simulink model "KFPID"  (R2015a)
settings: Solver=ode4  StartTime=0.0  StopTime=10.0  FixedStep=0.01  RelTol=1e-3
libraries: simulink x4
settings Model: Creator=LAB425  LastModifiedBy=LAB425

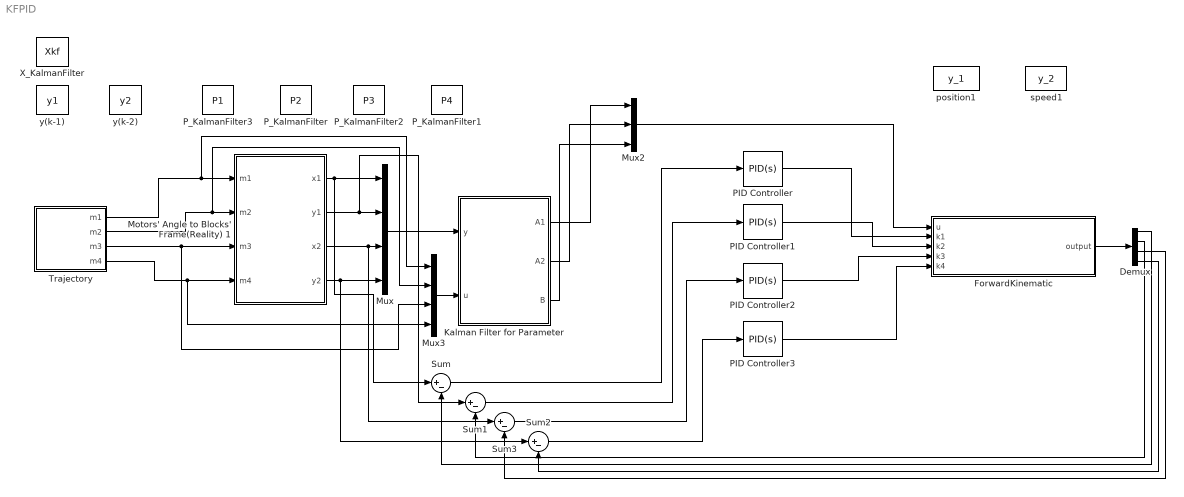
== system KFPID ==
  Demux : Demux
  ForwardKinematic : MATLAB Function  TreatAsAtomicUnit=on
  Kalman Filter for Parameter : MATLAB Function  TreatAsAtomicUnit=on
  Motors' Angle to Blocks' Frame(Reality) 1 : MATLAB Function  TreatAsAtomicUnit=on
  Mux : Mux
  Mux2 : Mux  Inputs=3
  Mux3 : Mux
  PID Controller{,1..3} (4 alike) : simulink/Continuous/PID Controller  Controller=PID  TimeDomain=Continuous-time  SampleTime=-1  IntegratorMethod=Forward Euler  FilterMethod=Forward Euler  Form=Parallel  UseFilter=on  ControllerParametersSource=internal  P=1  I=1  D=0  N=100  InitialConditionSource=internal  InitialConditionForIntegrator=0  InitialConditionForFilter=0  ExternalReset=none  LimitOutput=off  UpperSaturationLimit=inf  LowerSaturationLimit=-inf  LinearizeAsGain=on  AntiWindupMode=none  Kb=1  TrackingMode=off  Kt=1  PParamMin=[]  PParamMax=[]  IParamMin=[]  IParamMax=[]  DParamMin=[]  DParamMax=[]  NParamMin=[]  NParamMax=[]  KbParamMin=[]  KbParamMax=[]  KtParamMin=[]  KtParamMax=[]  POutMin=[]  POutMax=[]  IOutMin=[]  IOutMax=[]  DOutMin=[]  DOutMax=[]  NOutMin=[]  NOutMax=[]  KbOutMin=[]  KbOutMax=[]  KtOutMin=[]  KtOutMax=[]  IntegratorOutMin=[]  IntegratorOutMax=[]  FilterOutMin=[]  FilterOutMax=[]  SumOutMin=[]  SumOutMax=[]  SumI1OutMin=[]  SumI1OutMax=[]  SumI2OutMin=[]  SumI2OutMax=[]  SumI3OutMin=[]  SumI3OutMax=[]  SumDOutMin=[]  SumDOutMax=[]  SaturationOutMin=[]  SaturationOutMax=[]  IntegratorContinuousStateAttributes=''  IntegratorStateMustResolveToSignalObject=off  IntegratorRTWStateStorageClass=Auto  FilterContinuousStateAttributes=''  FilterStateMustResolveToSignalObject=off  FilterRTWStateStorageClass=Auto  DifferentiatorICPrevScaledInput=0  DifferentiatorOutMin=[]  DifferentiatorOutMax=[]
  P_KalmanFilter : DataStoreMemory  DataStoreName=P2  ReadBeforeWriteMsg=warning  WriteAfterWriteMsg=warning  WriteAfterReadMsg=warning  InitialValue=[0.001,0,0;0,0.002,0;0,0,0.001]  OutDataTypeStr=double
  P_KalmanFilter1 : DataStoreMemory  DataStoreName=P4  ReadBeforeWriteMsg=warning  WriteAfterWriteMsg=warning  WriteAfterReadMsg=warning  InitialValue=[0.001,0,0;0,0.002,0;0,0,0.001]  OutDataTypeStr=double
  P_KalmanFilter2 : DataStoreMemory  DataStoreName=P3  ReadBeforeWriteMsg=warning  WriteAfterWriteMsg=warning  WriteAfterReadMsg=warning  InitialValue=[0.001,0,0;0,0.002,0;0,0,0.001]  OutDataTypeStr=double
  P_KalmanFilter3 : DataStoreMemory  DataStoreName=P1  ReadBeforeWriteMsg=warning  WriteAfterWriteMsg=warning  WriteAfterReadMsg=warning  InitialValue=[0.001,0,0;0,0.002,0;0,0,0.001]  OutDataTypeStr=double
  Sum{,1..3} (4 alike) : Sum  Inputs=|+-
  Trajectory : Subsystem
  X_KalmanFilter : DataStoreMemory  DataStoreName=Xkf  ReadBeforeWriteMsg=warning  WriteAfterWriteMsg=warning  WriteAfterReadMsg=warning  InitialValue=[0,0,0,0;0,0,0,0;0,0,0,0]  OutDataTypeStr=double
  position1 : DataStoreMemory  DataStoreName=y_1  ReadBeforeWriteMsg=warning  WriteAfterWriteMsg=warning  WriteAfterReadMsg=warning  InitialValue=[0,0,0,0]  OutDataTypeStr=double
  speed1 : DataStoreMemory  DataStoreName=y_2  ReadBeforeWriteMsg=warning  WriteAfterWriteMsg=warning  WriteAfterReadMsg=warning  InitialValue=[0,0,0,0]  OutDataTypeStr=double
  y(k-1) : DataStoreMemory  DataStoreName=y1  ReadBeforeWriteMsg=warning  WriteAfterWriteMsg=warning  WriteAfterReadMsg=warning  InitialValue=[0,0,0,0]  OutDataTypeStr=double
  y(k-2) : DataStoreMemory  DataStoreName=y2  ReadBeforeWriteMsg=warning  WriteAfterWriteMsg=warning  WriteAfterReadMsg=warning  InitialValue=[0,0,0,0]  OutDataTypeStr=double
  wires:
  Motors' Angle to Blocks' Frame(Reality) 1/2(y1) -> Mux/2, Sum1/1
  Motors' Angle to Blocks' Frame(Reality) 1/3(x2) -> Sum3/1, Mux/3
  Motors' Angle to Blocks' Frame(Reality) 1/4(y2) -> Mux/4, Sum2/1
  Motors' Angle to Blocks' Frame(Reality) 1/1(x1) -> Mux/1, Sum/1
  Mux/1 -> Kalman Filter for Parameter/1(y)
  Mux3/1 -> Kalman Filter for Parameter/2(u)
  Trajectory/3(m3) -> Motors' Angle to Blocks' Frame(Reality) 1/3(m3), Mux3/3
  Trajectory/2(m2) -> Mux3/2, Motors' Angle to Blocks' Frame(Reality) 1/2(m2)
  Trajectory/4(m4) -> Motors' Angle to Blocks' Frame(Reality) 1/4(m4), Mux3/4
  Trajectory/1(m1) -> Mux3/1, Motors' Angle to Blocks' Frame(Reality) 1/1(m1)
  PID Controller/1 -> ForwardKinematic/2(k1)
  PID Controller1/1 -> ForwardKinematic/3(k2)
  PID Controller2/1 -> ForwardKinematic/4(k3)
  PID Controller3/1 -> ForwardKinematic/5(k4)
  Kalman Filter for Parameter/1(A1) -> Mux2/1
  Kalman Filter for Parameter/2(A2) -> Mux2/2
  Kalman Filter for Parameter/3(B) -> Mux2/3
  Sum/1 -> PID Controller/1
  Sum1/1 -> PID Controller1/1
  Sum3/1 -> PID Controller2/1
  Sum2/1 -> PID Controller3/1
  ForwardKinematic/1(output) -> Demux/1
  Demux/1 -> Sum/2
  Demux/2 -> Sum1/2
  Demux/3 -> Sum3/2
  Demux/4 -> Sum2/2
  Mux2/1 -> ForwardKinematic/1(u)

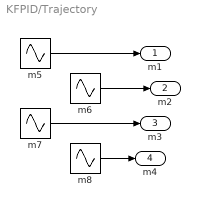
== system KFPID/Trajectory ==
  m5 : Sin  SampleTime=0
  m6 : Sin  Frequency=2  SampleTime=0
  m7 : Sin  Phase=3.14  SampleTime=0
  m8 : Sin  Frequency=2  Phase=3.14  SampleTime=0
  m1 : Outport
  m2 : Outport  Port=2
  m3 : Outport  Port=3
  m4 : Outport  Port=4
  wires:
  m6/1 -> m2/1
  m5/1 -> m1/1
  m7/1 -> m3/1
  m8/1 -> m4/1

== matlab function KFPID/Motors' Angle to Blocks' Frame(Reality) 1 ==
  data: x1 output; m1 input; y1 output; x2 output; m2 input; m3 input; m4 input; y2 output
function [x1,y1,x2,y2] = Signal(m1,m2,m3,m4)



%m1,m2,m3,m4为四个电机的当前时刻的角度值

%最远距离
D = 1.8;
% %螺距
% n = 0.02;
% %最大圈数
% ratio = D / n;
v=sqrt(0.0025)*randn(4,1);
x1 = m1 * D;
y1 = m2 * D;
x2 = m3 * D;
y2 = m4 * D;

if x1>=2
    x1=2;
else
    if x1<=-2
        x1=-2;
    end
end
if x2>=2
    x2=2;
else
    if x2<=-2
        x2=-2;
    end
end
if y1>=2
    y1=2;
else
    if y1<=-2
        y1=-2;
    end
end
if y2>=2
    y2=2;
else
    if y2<=-2
        y2=-2;
    end
end

== matlab function KFPID/Kalman Filter for Parameter ==
  data: y input; A1 output; u input; A2 output; B output; y1 data_store_memory; y2 data_store_memory; Xkf data_store_memory; P1 data_store_memory; P2 data_store_memory; P3 data_store_memory; P4 data_store_memory
function [A1,A2,B] = KalmanFilter(y,u)
global y1 y2 Xkf P1 P2 P3 P4
%% 单值参数识别（范例）
P = zeros(3,3,4);
P(:,:,1) = P1;
P(:,:,2) = P2;
P(:,:,3) = P3;
P(:,:,4) = P4;
Q = zeros(3,3);%过程噪声方差
R = 0.0001;%测量噪声方差
F = 1;%状态转移矩阵
for i = 1:1:4
    H = [y1(i) y2(i) u(i)];%1x3
    Z = y(i) + sqrt(R) * randn(1);
    X_pre = F * Xkf(:,i);%3x1
    P_pre = F * P(:,:,i) * F' + Q;%3x3
    Kg = P_pre * H' * inv(H * P_pre * H' + R);%3x1
    Xkf(:,i) = X_pre + Kg * (Z - H * X_pre); %3x1
    P(:,:,i) = (eye(3,3) - Kg * H) * P_pre;
end
P1 = P(:,:,1);
P2 = P(:,:,2);
P3 = P(:,:,3);
P4 = P(:,:,4);

y2 = y1;
y1 = y;%[x1,y1,x2,y2]
A1 = Xkf(1,:)';A2 = Xkf(2,:)'; B = Xkf(3,:)';

%A1:a1的四个电机参数
%A2:a2的四个电机参数
%B:b的四个电机参数

== matlab function KFPID/ForwardKinematic ==
  data: output output; u input; y_1 data_store_memory; y_2 data_store_memory; k1 input; k2 input; k3 input; k4 input
function output = RobotForwardKinematic(u,k1,k2,k3,k4) %输入1x4
global y_1 y_2
%% 单电机状态方程
param = u;
A = [0 1 0 0 0 0 0 0;
     -param(5) -param(1) 0 0 0 0 0 0;
     0 0 0 1 0 0 0 0;
     0 0 -param(6) -param(2) 0 0 0 0;
     0 0 0 0 0 1 0 0;
     0 0 0 0 -param(7) -param(3) 0 0;
     0 0 0 0 0 0 0 1;
     0 0 0 0 0 0 -param(8) -param(4)]; %8x8
b = [0 0 0 0;
     param(9) 0 0 0;
     0 0 0 0;
     0 param(10) 0 0;
     0 0 0 0;
     0 0 param(11) 0;
     0 0 0 0;
     0 0 0 param(12)]; % 8x4
C = [0 1 0 0 0 0 0 0;
     0 0 0 1 0 0 0 0;
     0 0 0 0 0 1 0 0;
     0 0 0 0 0 0 0 1];
% output = C * (A * x + b * u(13:16));
y = [y_2(1);y_1(1);y_2(2);y_1(2);y_2(3);y_1(3);y_2(4);y_1(4)];
x = y;
v=sqrt(0.001)*randn(4,1);
output = C * (A * x + b * [k1;k2;k3;k4]) ;
y_2 = y_1;
y_1 = output;
%%
